simulink model "Auto_mode"  (R2016a)
settings: Solver=VariableStepAuto  StartTime=0.0  StopTime=50  FixedStep=Ts  RelTol=1e-3
model workspace (MAT data in the model file):
  AC_ATTITUDE_ACCEL_Y_CONTROLLER_MAX_RADSS = Simulink.Signal
  AC_ATTITUDE_ACCEL_Y_CONTROLLER_MAX_RADSS.DataType = 'double'
  AC_ATTITUDE_ACCEL_Y_CONTROLLER_MAX_RADSS.Dimensions = 1
  AC_ATTITUDE_ACCEL_Y_CONTROLLER_MAX_RADSS.DimensionsMode = 'auto'
  AC_ATTITUDE_ACCEL_Y_CONTROLLER_MAX_RADSS.Complexity = 'real'
  AC_ATTITUDE_ACCEL_Y_CONTROLLER_MAX_RADSS.SampleTime = -1
  AC_ATTITUDE_ACCEL_Y_CONTROLLER_MAX_RADSS.SamplingMode = 'Sample based'
  AC_ATTITUDE_ACCEL_Y_CONTROLLER_MAX_RADSS.InitialValue = '0.5'
  AC_ATTITUDE_CONTROL_MAX = Simulink.Signal
  AC_ATTITUDE_CONTROL_MAX.DataType = 'double'
  AC_ATTITUDE_CONTROL_MAX.Dimensions = 1
  AC_ATTITUDE_CONTROL_MAX.DimensionsMode = 'auto'
  AC_ATTITUDE_CONTROL_MAX.Complexity = 'real'
  AC_ATTITUDE_CONTROL_MAX.SampleTime = -1
  AC_ATTITUDE_CONTROL_MAX.SamplingMode = 'Sample based'
  AC_ATTITUDE_CONTROL_MAX.InitialValue = '0.5'
  AC_ATTITUDE_THRUST_ERROR_ANGLE = Simulink.Signal
  AC_ATTITUDE_THRUST_ERROR_ANGLE.DataType = 'double'
  AC_ATTITUDE_THRUST_ERROR_ANGLE.Dimensions = 1
  AC_ATTITUDE_THRUST_ERROR_ANGLE.DimensionsMode = 'auto'
  AC_ATTITUDE_THRUST_ERROR_ANGLE.Complexity = 'real'
  AC_ATTITUDE_THRUST_ERROR_ANGLE.SampleTime = -1
  AC_ATTITUDE_THRUST_ERROR_ANGLE.SamplingMode = 'Sample based'
  AC_ATTITUDE_THRUST_ERROR_ANGLE.InitialValue = '1000'
  ROLL_PITCH_INPUT_MAX = Simulink.Signal
  ROLL_PITCH_INPUT_MAX.DataType = 'double'
  ROLL_PITCH_INPUT_MAX.Dimensions = 1
  ROLL_PITCH_INPUT_MAX.DimensionsMode = 'auto'
  ROLL_PITCH_INPUT_MAX.Complexity = 'real'
  ROLL_PITCH_INPUT_MAX.SampleTime = -1
  ROLL_PITCH_INPUT_MAX.SamplingMode = 'Sample based'
  ROLL_PITCH_INPUT_MAX.InitialValue = '3000'
  Sig = Simulink.Signal
  Sig.DataType = 'auto'
  Sig.Dimensions = -1
  Sig.DimensionsMode = 'auto'
  Sig.Complexity = 'auto'
  Sig.SampleTime = -1
  Sig.SamplingMode = 'auto'
  Sig1 = Simulink.Signal
  Sig1.DataType = 'auto'
  Sig1.Dimensions = -1
  Sig1.DimensionsMode = 'auto'
  Sig1.Complexity = 'auto'
  Sig1.SampleTime = -1
  Sig1.SamplingMode = 'auto'
  acro_yaw_p = Simulink.Signal
  acro_yaw_p.DataType = 'double'
  acro_yaw_p.Dimensions = 1
  acro_yaw_p.DimensionsMode = 'auto'
  acro_yaw_p.Complexity = 'real'
  acro_yaw_p.SampleTime = -1
  acro_yaw_p.SamplingMode = 'Sample based'
  acro_yaw_p.InitialValue = '45'
  angle_max = Simulink.Signal
  angle_max.DataType = 'double'
  angle_max.Dimensions = 1
  angle_max.DimensionsMode = 'auto'
  angle_max.Complexity = 'real'
  angle_max.SampleTime = -1
  angle_max.SamplingMode = 'Sample based'
  angle_max.InitialValue = '3000'
  attitude_target_ang_vel = Simulink.Signal
  attitude_target_ang_vel.DataType = 'double'
  attitude_target_ang_vel.Dimensions = 3
  attitude_target_ang_vel.DimensionsMode = 'auto'
  attitude_target_ang_vel.Complexity = 'real'
  attitude_target_ang_vel.SampleTime = -1
  attitude_target_ang_vel.SamplingMode = 'Sample based'
  attitude_target_ang_vel.InitialValue = '[0 0 0]'
  attitude_target_euler_angle_x = Simulink.Signal
  attitude_target_euler_angle_x.DataType = 'double'
  attitude_target_euler_angle_x.Dimensions = 1
  attitude_target_euler_angle_x.DimensionsMode = 'auto'
  attitude_target_euler_angle_x.Complexity = 'real'
  attitude_target_euler_angle_x.SampleTime = -1
  attitude_target_euler_angle_x.SamplingMode = 'Sample based'
  attitude_target_euler_angle_x.InitialValue = '0'
  attitude_target_euler_angle_y = Simulink.Signal
  attitude_target_euler_angle_y.DataType = 'double'
  attitude_target_euler_angle_y.Dimensions = 1
  attitude_target_euler_angle_y.DimensionsMode = 'auto'
  attitude_target_euler_angle_y.Complexity = 'real'
  attitude_target_euler_angle_y.SampleTime = -1
  attitude_target_euler_angle_y.SamplingMode = 'Sample based'
  attitude_target_euler_angle_y.InitialValue = '0'
  attitude_target_euler_angle_z = Simulink.Signal
  attitude_target_euler_angle_z.DataType = 'double'
  attitude_target_euler_angle_z.Dimensions = 1
  attitude_target_euler_angle_z.DimensionsMode = 'auto'
  attitude_target_euler_angle_z.Complexity = 'real'
  attitude_target_euler_angle_z.SampleTime = -1
  attitude_target_euler_angle_z.SamplingMode = 'Sample based'
  attitude_target_euler_angle_z.InitialValue = '0'
  attitude_target_euler_rate = Simulink.Signal
  attitude_target_euler_rate.DataType = 'double'
  attitude_target_euler_rate.Dimensions = 3
  attitude_target_euler_rate.DimensionsMode = 'auto'
  attitude_target_euler_rate.Complexity = 'real'
  attitude_target_euler_rate.SampleTime = -1
  attitude_target_euler_rate.SamplingMode = 'Sample based'
  attitude_target_euler_rate.InitialValue = '[0 0 0]'
  attitude_target_quat = Simulink.Signal
  attitude_target_quat.DataType = 'double'
  attitude_target_quat.Dimensions = 4
  attitude_target_quat.DimensionsMode = 'auto'
  attitude_target_quat.Complexity = 'real'
  attitude_target_quat.SampleTime = -1
  attitude_target_quat.SamplingMode = 'Sample based'
  attitude_target_quat.InitialValue = '[1 0 0 0]'
  attitude_vehicle_quat = Simulink.Signal
  attitude_vehicle_quat.DataType = 'double'
  attitude_vehicle_quat.Dimensions = 4
  attitude_vehicle_quat.DimensionsMode = 'auto'
  attitude_vehicle_quat.Complexity = 'real'
  attitude_vehicle_quat.SampleTime = -1
  attitude_vehicle_quat.SamplingMode = 'Sample based'
  attitude_vehicle_quat.InitialValue = '[1 0 0 0]'
  dt = Simulink.Signal
  dt.DataType = 'double'
  dt.Dimensions = 1
  dt.DimensionsMode = 'auto'
  dt.Complexity = 'real'
  dt.SampleTime = -1
  dt.SamplingMode = 'Sample based'
  dt.InitialValue = '0.01'
  false = 0
  limit_roll_pitch = Simulink.Signal
  limit_roll_pitch.DataType = 'double'
  limit_roll_pitch.Dimensions = 1
  limit_roll_pitch.DimensionsMode = 'auto'
  limit_roll_pitch.Complexity = 'real'
  limit_roll_pitch.SampleTime = -1
  limit_roll_pitch.SamplingMode = 'Sample based'
  limit_roll_pitch.InitialValue = '0.0'
  limit_throttle_upper = Simulink.Signal
  limit_throttle_upper.DataType = 'logical'
  limit_throttle_upper.Dimensions = 1
  limit_throttle_upper.DimensionsMode = 'auto'
  limit_throttle_upper.Complexity = 'real'
  limit_throttle_upper.SampleTime = -1
  limit_throttle_upper.SamplingMode = 'Sample based'
  limit_throttle_upper.InitialValue = '0'
  limit_yaw = Simulink.Signal
  limit_yaw.DataType = 'double'
  limit_yaw.Dimensions = 1
  limit_yaw.DimensionsMode = 'auto'
  limit_yaw.Complexity = 'real'
  limit_yaw.SampleTime = -1
  limit_yaw.SamplingMode = 'Sample based'
  limit_yaw.InitialValue = '0'
  loop_rate = Simulink.Signal
  loop_rate.DataType = 'double'
  loop_rate.Dimensions = 1
  loop_rate.DimensionsMode = 'auto'
  loop_rate.Complexity = 'real'
  loop_rate.SampleTime = -1
  loop_rate.SamplingMode = 'Sample based'
  loop_rate.InitialValue = '100'
  pitch_attitude_kP = Simulink.Signal
  pitch_attitude_kP.DataType = 'double'
  pitch_attitude_kP.Dimensions = 1
  pitch_attitude_kP.DimensionsMode = 'auto'
  pitch_attitude_kP.Complexity = 'real'
  pitch_attitude_kP.SampleTime = -1
  pitch_attitude_kP.SamplingMode = 'Sample based'
  pitch_attitude_kP.InitialValue = '20'
  pitch_factor = Simulink.Signal
  pitch_factor.DataType = 'double'
  pitch_factor.Dimensions = 4
  pitch_factor.DimensionsMode = 'auto'
  pitch_factor.Complexity = 'real'
  pitch_factor.SampleTime = -1
  pitch_factor.SamplingMode = 'Sample based'
  pitch_factor.InitialValue = '[cos(deg2rad(15)) -cos(deg2rad(15)) cos(deg2rad(15)) -cos(deg2rad(15))]'
  pitch_rate_derivative = Simulink.Signal
  pitch_rate_derivative.DataType = 'double'
  pitch_rate_derivative.Dimensions = 1
  pitch_rate_derivative.DimensionsMode = 'auto'
  pitch_rate_derivative.Complexity = 'real'
  pitch_rate_derivative.SampleTime = -1
  pitch_rate_derivative.SamplingMode = 'Sample based'
  pitch_rate_derivative.InitialValue = '0'
  pitch_rate_error_rads = Simulink.Signal
  pitch_rate_error_rads.DataType = 'double'
  pitch_rate_error_rads.Dimensions = 1
  pitch_rate_error_rads.DimensionsMode = 'auto'
  pitch_rate_error_rads.Complexity = 'real'
  pitch_rate_error_rads.SampleTime = -1
  pitch_rate_error_rads.SamplingMode = 'Sample based'
  pitch_rate_error_rads.InitialValue = '0'
  pitch_rate_filt_hz = Simulink.Signal
  pitch_rate_filt_hz.DataType = 'double'
  pitch_rate_filt_hz.Dimensions = 1
  pitch_rate_filt_hz.DimensionsMode = 'auto'
  pitch_rate_filt_hz.Complexity = 'real'
  pitch_rate_filt_hz.SampleTime = -1
  pitch_rate_filt_hz.SamplingMode = 'Sample based'
  pitch_rate_filt_hz.InitialValue = '1/(2*pi)'
  pitch_rate_imax = Simulink.Signal
  pitch_rate_imax.DataType = 'double'
  pitch_rate_imax.Dimensions = 1
  pitch_rate_imax.DimensionsMode = 'auto'
  pitch_rate_imax.Complexity = 'real'
  pitch_rate_imax.SampleTime = -1
  pitch_rate_imax.SamplingMode = 'Sample based'
  pitch_rate_imax.InitialValue = '200'
  pitch_rate_integrator = Simulink.Signal
  pitch_rate_integrator.DataType = 'double'
  pitch_rate_integrator.Dimensions = 1
  pitch_rate_integrator.DimensionsMode = 'auto'
  pitch_rate_integrator.Complexity = 'real'
  pitch_rate_integrator.SampleTime = -1
  pitch_rate_integrator.SamplingMode = 'Sample based'
  pitch_rate_integrator.InitialValue = '0'
  pitch_rate_kD = Simulink.Signal
  pitch_rate_kD.DataType = 'double'
  pitch_rate_kD.Dimensions = 1
  pitch_rate_kD.DimensionsMode = 'auto'
  pitch_rate_kD.Complexity = 'real'
  pitch_rate_kD.SampleTime = -1
  pitch_rate_kD.SamplingMode = 'Sample based'
  pitch_rate_kD.InitialValue = '0.004'
  pitch_rate_kI = Simulink.Signal
  pitch_rate_kI.DataType = 'double'
  pitch_rate_kI.Dimensions = 1
  pitch_rate_kI.DimensionsMode = 'auto'
  pitch_rate_kI.Complexity = 'real'
  pitch_rate_kI.SampleTime = -1
  pitch_rate_kI.SamplingMode = 'Sample based'
  pitch_rate_kI.InitialValue = '0.1'
  pitch_rate_kP = Simulink.Signal
  pitch_rate_kP.DataType = 'double'
  pitch_rate_kP.Dimensions = 1
  pitch_rate_kP.DimensionsMode = 'auto'
  pitch_rate_kP.Complexity = 'real'
  pitch_rate_kP.SampleTime = -1
  pitch_rate_kP.SamplingMode = 'Sample based'
  pitch_rate_kP.InitialValue = '0.5'
  pitch_rate_last_input = Simulink.Signal
  pitch_rate_last_input.DataType = 'double'
  pitch_rate_last_input.Dimensions = 1
  pitch_rate_last_input.DimensionsMode = 'auto'
  pitch_rate_last_input.Complexity = 'real'
  pitch_rate_last_input.SampleTime = -1
  pitch_rate_last_input.SamplingMode = 'Sample based'
  pitch_rate_last_input.InitialValue = '0'
  pitch_rate_proportional = Simulink.Signal
  pitch_rate_proportional.DataType = 'double'
  pitch_rate_proportional.Dimensions = 1
  pitch_rate_proportional.DimensionsMode = 'auto'
  pitch_rate_proportional.Complexity = 'real'
  pitch_rate_proportional.SampleTime = -1
  pitch_rate_proportional.SamplingMode = 'Sample based'
  pitch_rate_proportional.InitialValue = '0'
  pwm_max = Simulink.Signal
  pwm_max.DataType = 'double'
  pwm_max.Dimensions = 1
  pwm_max.DimensionsMode = 'auto'
  pwm_max.Complexity = 'real'
  pwm_max.SampleTime = -1
  pwm_max.SamplingMode = 'Sample based'
  pwm_max.InitialValue = '2000'
  pwm_min = Simulink.Signal
  pwm_min.DataType = 'double'
  pwm_min.Dimensions = 1
  pwm_min.DimensionsMode = 'auto'
  pwm_min.Complexity = 'real'
  pwm_min.SampleTime = -1
  pwm_min.SamplingMode = 'Sample based'
  pwm_min.InitialValue = '1039'
  rate_bf_ff_enabled = Simulink.Signal
  rate_bf_ff_enabled.DataType = 'double'
  rate_bf_ff_enabled.Dimensions = 1
  rate_bf_ff_enabled.DimensionsMode = 'auto'
  rate_bf_ff_enabled.Complexity = 'real'
  rate_bf_ff_enabled.SampleTime = -1
  rate_bf_ff_enabled.SamplingMode = 'Sample based'
  rate_bf_ff_enabled.InitialValue = '0'
  rate_target_ang_vel = Simulink.Signal
  rate_target_ang_vel.DataType = 'double'
  rate_target_ang_vel.Dimensions = 3
  rate_target_ang_vel.DimensionsMode = 'auto'
  rate_target_ang_vel.Complexity = 'real'
  rate_target_ang_vel.SampleTime = -1
  rate_target_ang_vel.SamplingMode = 'Sample based'
  rate_target_ang_vel.InitialValue = '[0 0 0]'
  roll_attitude_kP = Simulink.Signal
  roll_attitude_kP.DataType = 'double'
  roll_attitude_kP.Dimensions = 1
  roll_attitude_kP.DimensionsMode = 'auto'
  roll_attitude_kP.Complexity = 'real'
  roll_attitude_kP.SampleTime = -1
  roll_attitude_kP.SamplingMode = 'Sample based'
  roll_attitude_kP.InitialValue = '20'
  roll_factor = Simulink.Signal
  roll_factor.DataType = 'double'
  roll_factor.Dimensions = 4
  roll_factor.DimensionsMode = 'auto'
  roll_factor.Complexity = 'real'
  roll_factor.SampleTime = -1
  roll_factor.SamplingMode = 'Sample based'
  roll_factor.InitialValue = '[-sin(deg2rad(15)) sin(deg2rad(15)) sin(deg2rad(15)) -sin(deg2rad(15))]'
  roll_rate_derivative = Simulink.Signal
  roll_rate_derivative.DataType = 'double'
  roll_rate_derivative.Dimensions = 1
  roll_rate_derivative.DimensionsMode = 'auto'
  roll_rate_derivative.Complexity = 'real'
  roll_rate_derivative.SampleTime = -1
  roll_rate_derivative.SamplingMode = 'Sample based'
  roll_rate_derivative.InitialValue = '0'
  roll_rate_error_rads = Simulink.Signal
  roll_rate_error_rads.DataType = 'double'
  roll_rate_error_rads.Dimensions = 1
  roll_rate_error_rads.DimensionsMode = 'auto'
  roll_rate_error_rads.Complexity = 'real'
  roll_rate_error_rads.SampleTime = -1
  roll_rate_error_rads.SamplingMode = 'Sample based'
  roll_rate_error_rads.InitialValue = '0'
  roll_rate_filt_hz = Simulink.Signal
  roll_rate_filt_hz.DataType = 'double'
  roll_rate_filt_hz.Dimensions = 1
  roll_rate_filt_hz.DimensionsMode = 'auto'
  roll_rate_filt_hz.Complexity = 'real'
  roll_rate_filt_hz.SampleTime = -1
  roll_rate_filt_hz.SamplingMode = 'Sample based'
  roll_rate_filt_hz.InitialValue = '1/(2*pi)'
  roll_rate_imax = Simulink.Signal
  roll_rate_imax.DataType = 'double'
  roll_rate_imax.Dimensions = 1
  roll_rate_imax.DimensionsMode = 'auto'
  roll_rate_imax.Complexity = 'real'
  roll_rate_imax.SampleTime = -1
  roll_rate_imax.SamplingMode = 'Sample based'
  roll_rate_imax.InitialValue = '200'
  roll_rate_integrator = Simulink.Signal
  roll_rate_integrator.DataType = 'double'
  roll_rate_integrator.Dimensions = 1
  roll_rate_integrator.DimensionsMode = 'auto'
  roll_rate_integrator.Complexity = 'real'
  roll_rate_integrator.SampleTime = -1
  roll_rate_integrator.SamplingMode = 'Sample based'
  roll_rate_integrator.InitialValue = '0'
  roll_rate_kD = Simulink.Signal
  roll_rate_kD.DataType = 'double'
  roll_rate_kD.Dimensions = 1
  roll_rate_kD.DimensionsMode = 'auto'
  roll_rate_kD.Complexity = 'real'
  roll_rate_kD.SampleTime = -1
  roll_rate_kD.SamplingMode = 'Sample based'
  roll_rate_kD.InitialValue = '0.004'
  roll_rate_kI = Simulink.Signal
  roll_rate_kI.DataType = 'double'
  roll_rate_kI.Dimensions = 1
  roll_rate_kI.DimensionsMode = 'auto'
  roll_rate_kI.Complexity = 'real'
  roll_rate_kI.SampleTime = -1
  roll_rate_kI.SamplingMode = 'Sample based'
  roll_rate_kI.InitialValue = '0.1'
  roll_rate_kP = Simulink.Signal
  roll_rate_kP.DataType = 'double'
  roll_rate_kP.Dimensions = 1
  roll_rate_kP.DimensionsMode = 'auto'
  roll_rate_kP.Complexity = 'real'
  roll_rate_kP.SampleTime = -1
  roll_rate_kP.SamplingMode = 'Sample based'
  roll_rate_kP.InitialValue = '1'
  roll_rate_last_input = Simulink.Signal
  roll_rate_last_input.DataType = 'double'
  roll_rate_last_input.Dimensions = 1
  roll_rate_last_input.DimensionsMode = 'auto'
  roll_rate_last_input.Complexity = 'real'
  roll_rate_last_input.SampleTime = -1
  roll_rate_last_input.SamplingMode = 'Sample based'
  roll_rate_last_input.InitialValue = '0'
  roll_rate_proportional = Simulink.Signal
  roll_rate_proportional.DataType = 'double'
  roll_rate_proportional.Dimensions = 1
  roll_rate_proportional.DimensionsMode = 'auto'
  roll_rate_proportional.Complexity = 'real'
  roll_rate_proportional.SampleTime = -1
  roll_rate_proportional.SamplingMode = 'Sample based'
  roll_rate_proportional.InitialValue = '0'
  spin_max = Simulink.Signal
  spin_max.DataType = 'double'
  spin_max.Dimensions = 1
  spin_max.DimensionsMode = 'auto'
  spin_max.Complexity = 'real'
  spin_max.SampleTime = -1
  spin_max.SamplingMode = 'Sample based'
  spin_max.InitialValue = '0.95'
  spin_min = Simulink.Signal
  spin_min.DataType = 'double'
  spin_min.Dimensions = 1
  spin_min.DimensionsMode = 'auto'
  spin_min.Complexity = 'real'
  spin_min.SampleTime = -1
  spin_min.SamplingMode = 'Sample based'
  spin_min.InitialValue = '0.15'
  throttle_avg_max = Simulink.Signal
  throttle_avg_max.DataType = 'double'
  throttle_avg_max.Dimensions = 1
  throttle_avg_max.DimensionsMode = 'auto'
  throttle_avg_max.Complexity = 'real'
  throttle_avg_max.SampleTime = -1
  throttle_avg_max.SamplingMode = 'Sample based'
  throttle_avg_max.InitialValue = '0'
  throttle_filter_cutoff_freq = Simulink.Signal
  throttle_filter_cutoff_freq.DataType = 'double'
  throttle_filter_cutoff_freq.Dimensions = 1
  throttle_filter_cutoff_freq.DimensionsMode = 'auto'
  throttle_filter_cutoff_freq.Complexity = 'real'
  throttle_filter_cutoff_freq.SampleTime = -1
  throttle_filter_cutoff_freq.SamplingMode = 'Sample based'
  throttle_filter_cutoff_freq.InitialValue = '0.5'
  throttle_filter_output = Simulink.Signal
  throttle_filter_output.DataType = 'double'
  throttle_filter_output.Dimensions = 1
  throttle_filter_output.DimensionsMode = 'auto'
  throttle_filter_output.Complexity = 'real'
  throttle_filter_output.SampleTime = -1
  throttle_filter_output.SamplingMode = 'Sample based'
  throttle_filter_output.InitialValue = '0'
  throttle_in = Simulink.Signal
  throttle_in.DataType = 'double'
  throttle_in.Dimensions = 1
  throttle_in.DimensionsMode = 'auto'
  throttle_in.Complexity = 'real'
  throttle_in.SampleTime = -1
  throttle_in.SamplingMode = 'Sample based'
  throttle_in.InitialValue = '0'
  throttle_rpy_mix = Simulink.Signal
  throttle_rpy_mix.DataType = 'double'
  throttle_rpy_mix.Dimensions = 1
  throttle_rpy_mix.DimensionsMode = 'auto'
  throttle_rpy_mix.Complexity = 'real'
  throttle_rpy_mix.SampleTime = -1
  throttle_rpy_mix.SamplingMode = 'Sample based'
  throttle_rpy_mix.InitialValue = '0'
  throttle_rpy_mix_desired = Simulink.Signal
  throttle_rpy_mix_desired.DataType = 'double'
  throttle_rpy_mix_desired.Dimensions = 1
  throttle_rpy_mix_desired.DimensionsMode = 'auto'
  throttle_rpy_mix_desired.Complexity = 'real'
  throttle_rpy_mix_desired.SampleTime = -1
  throttle_rpy_mix_desired.SamplingMode = 'Sample based'
  throttle_rpy_mix_desired.InitialValue = '0'
  throttle_thrust = Simulink.Signal
  throttle_thrust.DataType = 'double'
  throttle_thrust.Dimensions = 1
  throttle_thrust.DimensionsMode = 'auto'
  throttle_thrust.Complexity = 'real'
  throttle_thrust.SampleTime = -1
  throttle_thrust.SamplingMode = 'Sample based'
  throttle_thrust.InitialValue = '0'
  throttle_thrust_best_rpy = Simulink.Signal
  throttle_thrust_best_rpy.DataType = 'double'
  throttle_thrust_best_rpy.Dimensions = 1
  throttle_thrust_best_rpy.DimensionsMode = 'auto'
  throttle_thrust_best_rpy.Complexity = 'real'
  throttle_thrust_best_rpy.SampleTime = -1
  throttle_thrust_best_rpy.SamplingMode = 'Sample based'
  throttle_thrust_best_rpy.InitialValue = '0'
  throttle_thrust_max = Simulink.Signal
  throttle_thrust_max.DataType = 'double'
  throttle_thrust_max.Dimensions = 1
  throttle_thrust_max.DimensionsMode = 'auto'
  throttle_thrust_max.Complexity = 'real'
  throttle_thrust_max.SampleTime = -1
  throttle_thrust_max.SamplingMode = 'Sample based'
  throttle_thrust_max.InitialValue = '1'
  thrust_error_angle = Simulink.Signal
  thrust_error_angle.DataType = 'double'
  thrust_error_angle.Dimensions = 1
  thrust_error_angle.DimensionsMode = 'auto'
  thrust_error_angle.Complexity = 'real'
  thrust_error_angle.SampleTime = -1
  thrust_error_angle.SamplingMode = 'Sample based'
  thrust_error_angle.InitialValue = '0'
  thrust_rpyt_out = Simulink.Signal
  thrust_rpyt_out.DataType = 'double'
  thrust_rpyt_out.Dimensions = 4
  thrust_rpyt_out.DimensionsMode = 'auto'
  thrust_rpyt_out.Complexity = 'real'
  thrust_rpyt_out.SampleTime = -1
  thrust_rpyt_out.SamplingMode = 'Sample based'
  thrust_rpyt_out.InitialValue = '[0 0 0 0]'
  true = 1
  use_ff_and_input_shaping = Simulink.Signal
  use_ff_and_input_shaping.DataType = 'double'
  use_ff_and_input_shaping.Dimensions = 1
  use_ff_and_input_shaping.DimensionsMode = 'auto'
  use_ff_and_input_shaping.Complexity = 'real'
  use_ff_and_input_shaping.SampleTime = -1
  use_ff_and_input_shaping.SamplingMode = 'Sample based'
  use_ff_and_input_shaping.InitialValue = '0'
  variableType = 'S'
  yaw_allowed = Simulink.Signal
  yaw_allowed.DataType = 'double'
  yaw_allowed.Dimensions = 1
  yaw_allowed.DimensionsMode = 'auto'
  yaw_allowed.Complexity = 'real'
  yaw_allowed.SampleTime = -1
  yaw_allowed.SamplingMode = 'Sample based'
  yaw_allowed.InitialValue = '1'
  yaw_attitude_kP = Simulink.Signal
  yaw_attitude_kP.DataType = 'double'
  yaw_attitude_kP.Dimensions = 1
  yaw_attitude_kP.DimensionsMode = 'auto'
  yaw_attitude_kP.Complexity = 'real'
  yaw_attitude_kP.SampleTime = -1
  yaw_attitude_kP.SamplingMode = 'Sample based'
  yaw_attitude_kP.InitialValue = '4.5'
  yaw_factor = Simulink.Signal
  yaw_factor.DataType = 'double'
  yaw_factor.Dimensions = 4
  yaw_factor.DimensionsMode = 'auto'
  yaw_factor.Complexity = 'real'
  yaw_factor.SampleTime = -1
  yaw_factor.SamplingMode = 'Sample based'
  yaw_factor.InitialValue = '[0.1 0.1 -0.1 -0.1]'
  yaw_headroom = Simulink.Signal
  yaw_headroom.DataType = 'double'
  yaw_headroom.Dimensions = 1
  yaw_headroom.DimensionsMode = 'auto'
  yaw_headroom.Complexity = 'real'
  yaw_headroom.SampleTime = -1
  yaw_headroom.SamplingMode = 'Sample based'
  yaw_headroom.InitialValue = '200'
  yaw_rate_derivative = Simulink.Signal
  yaw_rate_derivative.DataType = 'double'
  yaw_rate_derivative.Dimensions = 1
  yaw_rate_derivative.DimensionsMode = 'auto'
  yaw_rate_derivative.Complexity = 'real'
  yaw_rate_derivative.SampleTime = -1
  yaw_rate_derivative.SamplingMode = 'Sample based'
  yaw_rate_derivative.InitialValue = '0'
  yaw_rate_error_rads = Simulink.Signal
  yaw_rate_error_rads.DataType = 'double'
  yaw_rate_error_rads.Dimensions = 1
  yaw_rate_error_rads.DimensionsMode = 'auto'
  yaw_rate_error_rads.Complexity = 'real'
  yaw_rate_error_rads.SampleTime = -1
  yaw_rate_error_rads.SamplingMode = 'Sample based'
  yaw_rate_error_rads.InitialValue = '0'
  yaw_rate_filt_hz = Simulink.Signal
  yaw_rate_filt_hz.DataType = 'double'
  yaw_rate_filt_hz.Dimensions = 1
  yaw_rate_filt_hz.DimensionsMode = 'auto'
  yaw_rate_filt_hz.Complexity = 'real'
  yaw_rate_filt_hz.SampleTime = -1
  yaw_rate_filt_hz.SamplingMode = 'Sample based'
  yaw_rate_filt_hz.InitialValue = '1/(2*pi)'
  yaw_rate_imax = Simulink.Signal
  yaw_rate_imax.DataType = 'double'
  yaw_rate_imax.Dimensions = 1
  yaw_rate_imax.DimensionsMode = 'auto'
  yaw_rate_imax.Complexity = 'real'
  yaw_rate_imax.SampleTime = -1
  yaw_rate_imax.SamplingMode = 'Sample based'
  yaw_rate_imax.InitialValue = '200'
  yaw_rate_integrator = Simulink.Signal
  yaw_rate_integrator.DataType = 'double'
  yaw_rate_integrator.Dimensions = 1
  yaw_rate_integrator.DimensionsMode = 'auto'
  yaw_rate_integrator.Complexity = 'real'
  yaw_rate_integrator.SampleTime = -1
  yaw_rate_integrator.SamplingMode = 'Sample based'
  yaw_rate_integrator.InitialValue = '0'
  yaw_rate_kD = Simulink.Signal
  yaw_rate_kD.DataType = 'double'
  yaw_rate_kD.Dimensions = 1
  yaw_rate_kD.DimensionsMode = 'auto'
  yaw_rate_kD.Complexity = 'real'
  yaw_rate_kD.SampleTime = -1
  yaw_rate_kD.SamplingMode = 'Sample based'
  yaw_rate_kD.InitialValue = '5'
  yaw_rate_kI = Simulink.Signal
  yaw_rate_kI.DataType = 'double'
  yaw_rate_kI.Dimensions = 1
  yaw_rate_kI.DimensionsMode = 'auto'
  yaw_rate_kI.Complexity = 'real'
  yaw_rate_kI.SampleTime = -1
  yaw_rate_kI.SamplingMode = 'Sample based'
  yaw_rate_kI.InitialValue = '0.1'
  yaw_rate_kP = Simulink.Signal
  yaw_rate_kP.DataType = 'double'
  yaw_rate_kP.Dimensions = 1
  yaw_rate_kP.DimensionsMode = 'auto'
  yaw_rate_kP.Complexity = 'real'
  yaw_rate_kP.SampleTime = -1
  yaw_rate_kP.SamplingMode = 'Sample based'
  yaw_rate_kP.InitialValue = '0.2'
  yaw_rate_last_input = Simulink.Signal
  yaw_rate_last_input.DataType = 'double'
  yaw_rate_last_input.Dimensions = 1
  yaw_rate_last_input.DimensionsMode = 'auto'
  yaw_rate_last_input.Complexity = 'real'
  yaw_rate_last_input.SampleTime = -1
  yaw_rate_last_input.SamplingMode = 'Sample based'
  yaw_rate_last_input.InitialValue = '0'
  yaw_rate_proportional = Simulink.Signal
  yaw_rate_proportional.DataType = 'double'
  yaw_rate_proportional.Dimensions = 1
  yaw_rate_proportional.DimensionsMode = 'auto'
  yaw_rate_proportional.Complexity = 'real'
  yaw_rate_proportional.SampleTime = -1
  yaw_rate_proportional.SamplingMode = 'Sample based'
  yaw_rate_proportional.InitialValue = '0'
undefined symbols (not defined in the file): Ts
libraries: aerolibactuator x2, vrlib x2, aerolib6dof2 x1, aerolibutil x1, aerolibconvert2 x1
settings Model: Creator=s121814  LastModifiedBy=GusBus
settings SolverCC: ZeroCrossControl=DisableAll
settings DataIOCC: SaveFormat=Array  SaveState=on

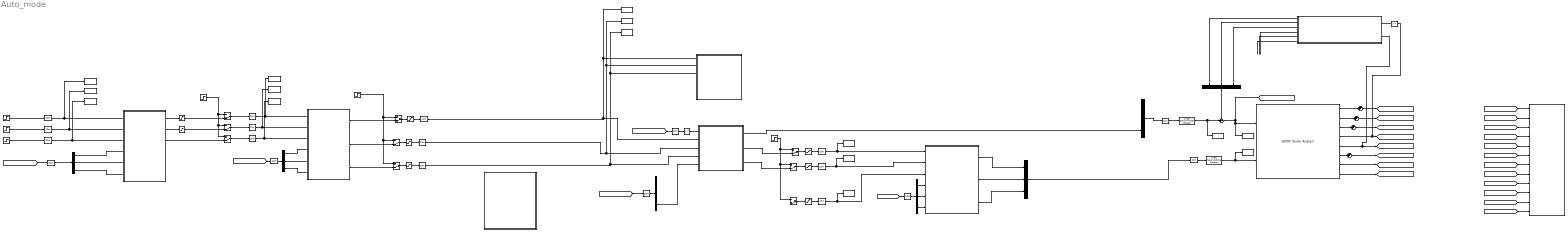
== system Auto_mode ==
  note: Step Response and Switches used for tuning
  Demux{,1..3} (4 alike) : Demux  Outputs=3
  Flight Kinematics : aerolib6dof2/6DOF (Euler Angles)  units=Metric (MKS)  mtype=Fixed  rep=Euler Angles  xme_0=[0 0 0]  Vm_0=[0 0 0]  eul_0=[0 0 0]  pm_0=[0 0 0]  mass_0=3.352  mass_e=0.5  mass_f=2.0  inertia=[0.025028 0 0; 0 0.16926 0; 0 0 0.170197]  inertia_e=eye(3)  inertia_f=2*eye(3)  k_quat=1.0  vre_flag=on
  Gravity and Drag Distrubance Calculation : MATLAB Function  TreatAsAtomicUnit=on
  Linear Second-Order Actuator1 : aerolibactuator/Linear Second-Order Actuator  wn_fin=100  z_fin=1  fin_act_0=0  fin_act_vel=0
  Linear Second-Order Actuator2 : aerolibactuator/Linear Second-Order Actuator  wn_fin=100  z_fin=1  fin_act_0=0  fin_act_vel=0
  Linear Velocity Controller : Subsystem
  Manual Switch{,1..5,9..11} (9 alike) : ManualSwitch  CurrentSetting=0
  Math Function : Math  Operator=transpose  SaturateOnIntegerOverflow=on
  Math Function1 : Math  Operator=transpose  SaturateOnIntegerOverflow=on
  Position Controller : Subsystem
  Rate Controller : Subsystem
  Saturation : Saturate  UpperLimit=deg2rad(15)  LowerLimit=-deg2rad(15)
  Saturation1 : Saturate  UpperLimit=deg2rad(15)  LowerLimit=-deg2rad(15)
  Saturation2 : Saturate  UpperLimit=15  LowerLimit=-15
  Saturation3 : Saturate  UpperLimit=15  LowerLimit=-15
  Saturation4 : Saturate  UpperLimit=100  LowerLimit=-100
  Saturation5 : Saturate  UpperLimit=15  LowerLimit=-15
  Saturation6 : Saturate  UpperLimit=1  LowerLimit=-1
  Saturation7 : Saturate  UpperLimit=1  LowerLimit=-1
  Step : Step  Time=0  After=0  SampleTime=0
  Step1 : Step  Time=0  After=0  SampleTime=0
  Step2 : Step  After=0  SampleTime=0
  Step3 : Step  SampleTime=0
  Step5 : Step  After=0.18  SampleTime=0
  Step6 : Step  After=5  SampleTime=0
  Sum1 : Sum  Inputs=-+|
  Sum{5,7,9..10} (4 alike) : Sum  Inputs=++|
  Thrust Controller : Subsystem
  Tilt Angle Controller : Subsystem
  To Workspace and Graphics : Subsystem
  To Workspace1 : ToWorkspace  VariableName=refrollrate  SampleTime=-1
  To Workspace10 : ToWorkspace  VariableName=forces  SampleTime=-1
  To Workspace11 : ToWorkspace  VariableName=moments  SampleTime=-1
  To Workspace12 : ToWorkspace  VariableName=refxvel_e  SampleTime=-1
  To Workspace13 : ToWorkspace  VariableName=refyvel_e  SampleTime=-1
  To Workspace14 : ToWorkspace  VariableName=refzvel_e  SampleTime=-1
  To Workspace15 : ToWorkspace  VariableName=forces1  SampleTime=-1
  To Workspace2 : ToWorkspace  VariableName=refpitchrate  SampleTime=-1
  To Workspace3 : ToWorkspace  VariableName=refxaccel  SampleTime=-1
  To Workspace4 : ToWorkspace  VariableName=refyaccel  SampleTime=-1
  To Workspace5 : ToWorkspace  VariableName=refzaccel  SampleTime=-1
  To Workspace6 : ToWorkspace  VariableName=refyawrate  SampleTime=-1
  To Workspace7 : ToWorkspace  VariableName=refxpos  SampleTime=-1
  To Workspace8 : ToWorkspace  VariableName=refypos  SampleTime=-1
  To Workspace9 : ToWorkspace  VariableName=refzpos  SampleTime=-1
  Vector Concatenate1 : Concatenate  NumInputs=3
  Vector Concatenate2 : Concatenate  NumInputs=3
  Vector Concatenate7 : Concatenate  NumInputs=3
  Vector Rotation : Subsystem
  Zero-Order Hold{1..19} (19 alike) : ZeroOrderHold  SampleTime=Ts
  tag scope: body_forces=global, body_linear_acceleration=global, body_linear_velocity=global, body_rotational_acceleration=global, body_rotational_velocity=global, dcm_body_earth=global, earth_linear_position=global, earth_linear_velocity=global, euler_angles_rad=global
  wires:
  [body_rotational_velocity] -> To Workspace and Graphics/6(body_rotational_velocity)
  [body_linear_acceleration] -> To Workspace and Graphics/8(body_linear_acceleration)
  [body_rotational_acceleration] -> To Workspace and Graphics/7(body_rotational_acceleration)
  [body_linear_velocity] -> To Workspace and Graphics/5(body_linear_velocity)
  [dcm_body_earth] -> To Workspace and Graphics/4(dcm_body_earth)
  [euler_angles_rad] -> To Workspace and Graphics/3(euler_angles_rad)
  [earth_linear_position] -> To Workspace and Graphics/2(earth_linear_position)
  [earth_linear_velocity] -> To Workspace and Graphics/1(earth_linear_velocity)
  Sum7/1 -> [earth_linear_velocity]  "earth_linear_velocity"
  Flight Kinematics/7 -> [body_rotational_acceleration]  "body_rotational_acceleration"
  Flight Kinematics/8 -> [body_linear_acceleration]  "body_linear_acceleration"
  Vector Concatenate7/1 -> Zero-Order Hold5/1
  Sum10/1 -> [euler_angles_rad]
  Flight Kinematics/3 -> Sum10/2  "euler_angles_rad"
  Sum9/1 -> [earth_linear_position]
  Flight Kinematics/2 -> Sum9/2
  Flight Kinematics/6 -> Sum5/2  "body_rotational_velocity"
  Sum5/1 -> [body_rotational_velocity]
  Flight Kinematics/1 -> Sum7/2
  [earth_linear_position_est] -> To Workspace and Graphics/12(earth_linear_position_est)
  [earth_linear_velocity_est] -> To Workspace and Graphics/11(earth_linear_velocity_est)
  [body_rotational_velocity_est] -> To Workspace and Graphics/10(body_rotational_velocity_est)
  [euler_angles_rad_est] -> To Workspace and Graphics/9(euler_angles_rad_est)
  Rate Controller/1(Torque Phi) -> Vector Concatenate7/1
  Rate Controller/2(Torque Theta) -> Vector Concatenate7/2
  Rate Controller/3(Torque Psi) -> Vector Concatenate7/3
  Demux/1 -> Rate Controller/4(roll_rate_current)
  Demux/2 -> Rate Controller/5(pitch_rate_current)
  Demux/3 -> Rate Controller/6(yaw_rate_current)
  [body_rotational_velocity] -> Zero-Order Hold1/1
  Zero-Order Hold1/1 -> Demux/1
  Zero-Order Hold5/1 -> Linear Second-Order Actuator1/1
  Vector Concatenate1/1 -> Zero-Order Hold6/1
  Zero-Order Hold6/1 -> Linear Second-Order Actuator2/1
  Linear Second-Order Actuator1/1 -> To Workspace11/1, Flight Kinematics/2  "moments"
  Sum1/1 -> [body_forces], To Workspace10/1, Flight Kinematics/1  "Forces"
  Step/1 -> Zero-Order Hold2/1  "x_pos_target"
  Step2/1 -> Zero-Order Hold4/1  "z_pos_target"
  Step1/1 -> Zero-Order Hold3/1  "y_pos_target"
  Zero-Order Hold2/1 -> To Workspace7/1, Position Controller/1(x_pos_target)
  Zero-Order Hold3/1 -> To Workspace8/1, Position Controller/2(y_pos_target)
  Zero-Order Hold4/1 -> To Workspace9/1, Position Controller/3(z_pos_target)
  [earth_linear_position] -> Zero-Order Hold14/1
  Demux2/2 -> Position Controller/5(y_pos_current)
  Demux2/1 -> Position Controller/4(x_pos_current)
  Demux2/3 -> Position Controller/6(z_pos_current)
  Saturation/1 -> Zero-Order Hold8/1
  Saturation1/1 -> Zero-Order Hold9/1
  Saturation2/1 -> Zero-Order Hold19/1
  Saturation3/1 -> Zero-Order Hold18/1
  Saturation4/1 -> Zero-Order Hold17/1
  [dcm_body_earth] -> Zero-Order Hold16/1
  Saturation5/1 -> Zero-Order Hold10/1
  Zero-Order Hold14/1 -> Demux2/1
  Zero-Order Hold16/1 -> Math Function/1
  Step3/1 -> Manual Switch2/1, Manual Switch/1, Manual Switch1/1
  Manual Switch/1 -> Saturation3/1
  Manual Switch1/1 -> Saturation2/1
  Manual Switch2/1 -> Saturation4/1
  Linear Velocity Controller/1(x_accel_desired_earth) -> Manual Switch1/2
  Linear Velocity Controller/2(y_accel_desired_earth) -> Manual Switch/2
  Linear Velocity Controller/3(z_accel_desired_earth) -> Manual Switch2/2
  Tilt Angle Controller/3(desired_pitch_rate_rad/s) -> Manual Switch3/2
  Math Function/1 -> Tilt Angle Controller/1(dcm_eb)
  Step5/1 -> Manual Switch5/1, Manual Switch3/1, Manual Switch4/1
  Tilt Angle Controller/2(deired_roll_rate_rad/s) -> Manual Switch4/2
  Manual Switch4/1 -> Saturation/1
  Manual Switch3/1 -> Saturation1/1
  Manual Switch5/1 -> Saturation5/1
  Tilt Angle Controller/1(Z) -> Vector Concatenate1/3
  [earth_linear_velocity] -> Zero-Order Hold7/1
  Demux3/2 -> Linear Velocity Controller/5(y_vel_current_earth)
  Demux3/1 -> Linear Velocity Controller/4(x_vel_current_earth)
  Demux3/3 -> Linear Velocity Controller/6(z_vel_current_earth)
  Zero-Order Hold7/1 -> Demux3/1
  Manual Switch9/1 -> Zero-Order Hold12/1
  Manual Switch11/1 -> Zero-Order Hold13/1
  Manual Switch10/1 -> Zero-Order Hold11/1
  Zero-Order Hold11/1 -> Linear Velocity Controller/1(x_vel_target_earth), To Workspace12/1
  Zero-Order Hold13/1 -> Linear Velocity Controller/3(z_vel_target_earth), To Workspace14/1
  Position Controller/1(x_vel_desired_earth) -> Saturation6/1
  Position Controller/2(y_vel_desired_earth) -> Saturation7/1
  Step6/1 -> Manual Switch10/1, Manual Switch9/1, Manual Switch11/1
  Linear Second-Order Actuator2/1 -> To Workspace15/1, Sum1/2  "Forces"
  Gravity and Drag Distrubance Calculation/6(FDz) -> ?  "force_drag_z"
  Gravity and Drag Distrubance Calculation/2(FGy) -> Vector Concatenate2/2  "force_gravity_y"
  Flight Kinematics/4 -> Math Function1/1, [dcm_body_earth]  "dcm_body_earth"
  Gravity and Drag Distrubance Calculation/1(FGx) -> Vector Concatenate2/1  "force_gravity_x"
  Math Function1/1 -> Gravity and Drag Distrubance Calculation/1(DCMeb)
  Flight Kinematics/5 -> Gravity and Drag Distrubance Calculation/2(Vb), [body_linear_velocity]  "body_linear_velocity"
  Gravity and Drag Distrubance Calculation/3(FGz) -> Vector Concatenate2/3  "force_gravity_z"
  Gravity and Drag Distrubance Calculation/4(FDx) -> ?  "force_drag_x"
  Gravity and Drag Distrubance Calculation/5(FDy) -> ?  "force_drag_y"
  Vector Concatenate2/1 -> Sum1/1
  Saturation6/1 -> Manual Switch10/2
  Saturation7/1 -> Manual Switch9/2
  Position Controller/3(z_vel_desired_earth) -> Manual Switch11/2
  Zero-Order Hold8/1 -> To Workspace1/1, Rate Controller/1(roll_rate_target)
  Zero-Order Hold9/1 -> To Workspace2/1, Rate Controller/2(pitch_rate_target)
  Zero-Order Hold10/1 -> To Workspace6/1, Rate Controller/3(yaw_rate_target)
  Zero-Order Hold19/1 -> Thrust Controller/1(desired_accel_x_earth), To Workspace3/1, Tilt Angle Controller/2(desired_accel_x_earth)
  Zero-Order Hold18/1 -> Thrust Controller/2(desired_accel_y_earth), To Workspace4/1, Tilt Angle Controller/3(desired_accel_y_earth)
  Zero-Order Hold17/1 -> Thrust Controller/3(desired_accel_z_earth), To Workspace5/1, Tilt Angle Controller/4(desired_accel_z_earth)
  Zero-Order Hold12/1 -> Linear Velocity Controller/2(y_vel_target_earth), To Workspace13/1
  Demux1/3 -> Tilt Angle Controller/5(current_Z_Force)
  Zero-Order Hold15/1 -> Demux1/1
  [body_forces] -> Zero-Order Hold15/1

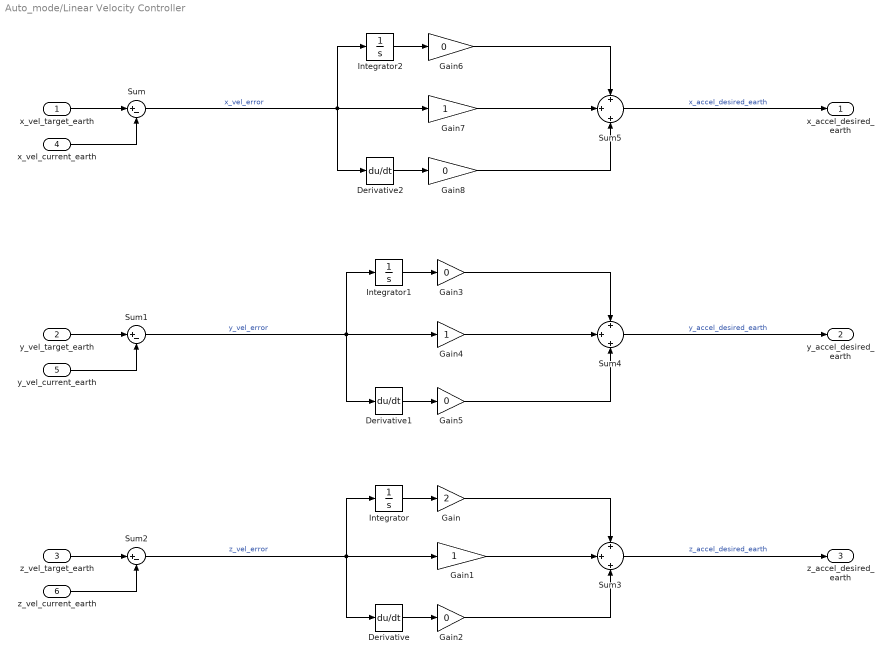
== system Auto_mode/Linear Velocity Controller ==
  x_vel_target_earth : Inport
  y_vel_target_earth : Inport  Port=2
  z_vel_target_earth : Inport  Port=3
  x_vel_current_earth : Inport  Port=4
  y_vel_current_earth : Inport  Port=5
  z_vel_current_earth : Inport  Port=6
  Derivative : Derivative
  Derivative1 : Derivative
  Derivative2 : Derivative
  Gain : Gain  Gain=2
  Gain1 : Gain
  Gain{2..3,5..6,8} (5 alike) : Gain  Gain=0
  Gain4 : Gain
  Gain7 : Gain
  Integrator : Integrator
  Integrator1 : Integrator
  Integrator2 : Integrator
  Sum : Sum  Inputs=|+-
  Sum1 : Sum  Inputs=|+-
  Sum2 : Sum  Inputs=|+-
  Sum3 : Sum  Inputs=+|+|+
  Sum4 : Sum  Inputs=+|+|+
  Sum5 : Sum  Inputs=+|+|+
  x_accel_desired_earth : Outport
  y_accel_desired_earth : Outport  Port=2
  z_accel_desired_earth : Outport  Port=3
  wires:
  x_vel_target_earth/1 -> Sum/1
  x_vel_current_earth/1 -> Sum/2
  y_vel_target_earth/1 -> Sum1/1
  y_vel_current_earth/1 -> Sum1/2
  z_vel_target_earth/1 -> Sum2/1
  z_vel_current_earth/1 -> Sum2/2
  Sum3/1 -> z_accel_desired_earth/1  "z_accel_desired_earth"
  Derivative/1 -> Gain2/1
  Gain2/1 -> Sum3/3
  Gain/1 -> Sum3/1
  Integrator/1 -> Gain/1
  Sum2/1 -> Integrator/1, Derivative/1, Gain1/1  "z_vel_error"
  Derivative1/1 -> Gain5/1
  Gain5/1 -> Sum4/3
  Gain4/1 -> Sum4/2
  Gain3/1 -> Sum4/1
  Integrator1/1 -> Gain3/1
  Sum1/1 -> Integrator1/1, Derivative1/1, Gain4/1  "y_vel_error"
  Sum4/1 -> y_accel_desired_earth/1  "y_accel_desired_earth"
  Derivative2/1 -> Gain8/1
  Gain8/1 -> Sum5/3
  Gain7/1 -> Sum5/2
  Gain6/1 -> Sum5/1
  Integrator2/1 -> Gain6/1
  Sum/1 -> Integrator2/1, Derivative2/1, Gain7/1  "x_vel_error"
  Sum5/1 -> x_accel_desired_earth/1  "x_accel_desired_earth"
  Gain1/1 -> Sum3/2

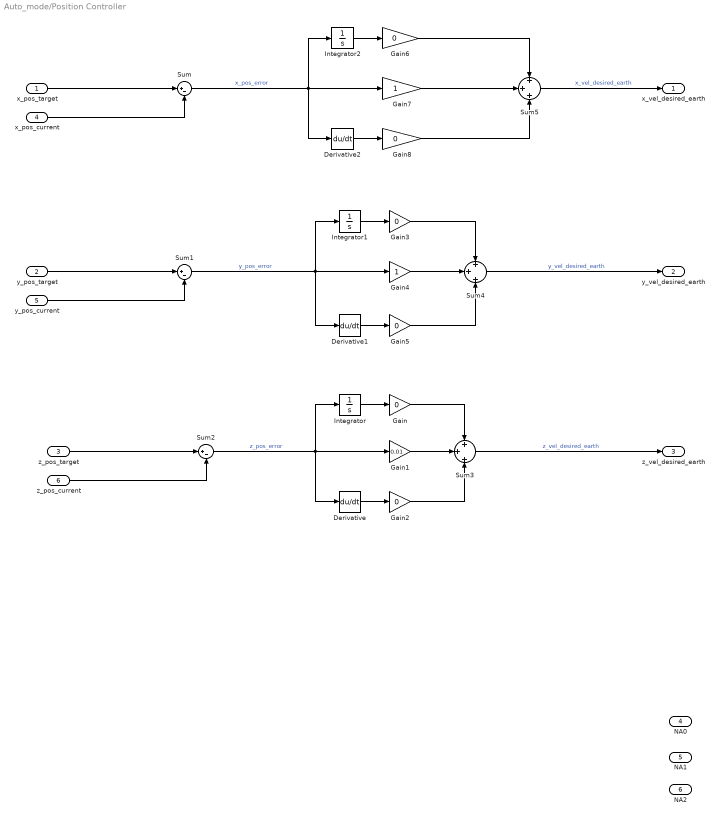
== system Auto_mode/Position Controller ==
  x_pos_target : Inport
  y_pos_target : Inport  Port=2
  z_pos_target : Inport  Port=3
  x_pos_current : Inport  Port=4
  y_pos_current : Inport  Port=5
  z_pos_current : Inport  Port=6
  Derivative : Derivative
  Derivative1 : Derivative
  Derivative2 : Derivative
  Gain{,2..3,5..6,8} (6 alike) : Gain  Gain=0
  Gain1 : Gain  Gain=0.01
  Gain4 : Gain
  Gain7 : Gain
  Integrator : Integrator
  Integrator1 : Integrator
  Integrator2 : Integrator
  Sum : Sum  Inputs=|+-
  Sum1 : Sum  Inputs=|+-
  Sum2 : Sum  Inputs=|+-
  Sum3 : Sum  Inputs=+|+|+
  Sum4 : Sum  Inputs=+|+|+
  Sum5 : Sum  Inputs=+|+|+
  x_vel_desired_earth : Outport
  y_vel_desired_earth : Outport  Port=2
  z_vel_desired_earth : Outport  Port=3
  NA0 : Outport  Port=4
  NA1 : Outport  Port=5
  NA2 : Outport  Port=6
  wires:
  x_pos_target/1 -> Sum/1
  x_pos_current/1 -> Sum/2
  y_pos_target/1 -> Sum1/1
  y_pos_current/1 -> Sum1/2
  z_pos_target/1 -> Sum2/1
  z_pos_current/1 -> Sum2/2
  Sum3/1 -> z_vel_desired_earth/1  "z_vel_desired_earth"
  Derivative/1 -> Gain2/1
  Gain2/1 -> Sum3/3
  Gain1/1 -> Sum3/2
  Gain/1 -> Sum3/1
  Integrator/1 -> Gain/1
  Sum2/1 -> Integrator/1, Derivative/1, Gain1/1  "z_pos_error"
  Derivative1/1 -> Gain5/1
  Gain5/1 -> Sum4/3
  Gain4/1 -> Sum4/2
  Gain3/1 -> Sum4/1
  Integrator1/1 -> Gain3/1
  Sum1/1 -> Integrator1/1, Derivative1/1, Gain4/1  "y_pos_error"
  Sum4/1 -> y_vel_desired_earth/1  "y_vel_desired_earth"
  Derivative2/1 -> Gain8/1
  Gain8/1 -> Sum5/3
  Gain7/1 -> Sum5/2
  Gain6/1 -> Sum5/1
  Integrator2/1 -> Gain6/1
  Sum/1 -> Integrator2/1, Derivative2/1, Gain7/1  "x_pos_error"
  Sum5/1 -> x_vel_desired_earth/1  "x_vel_desired_earth"

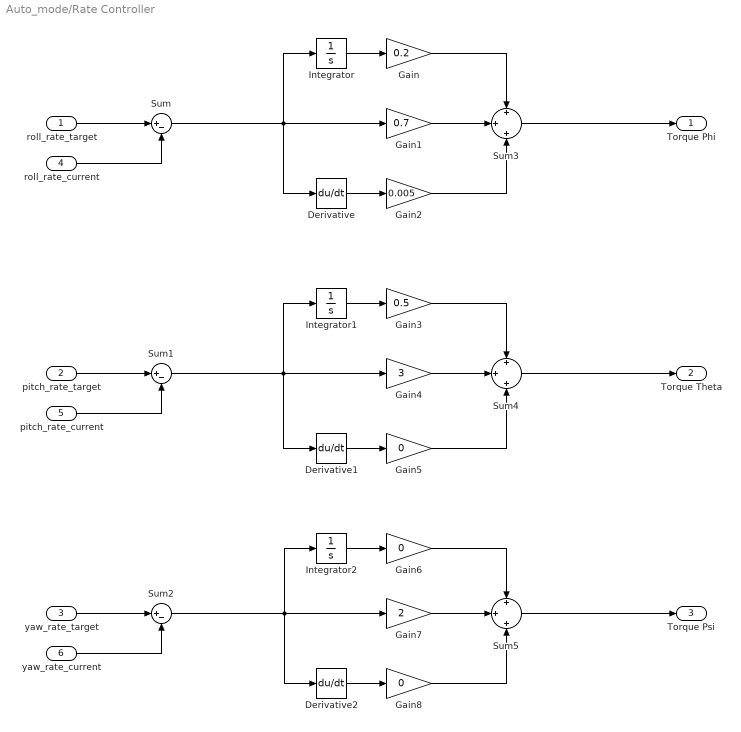
== system Auto_mode/Rate Controller ==
  roll_rate_target : Inport
  pitch_rate_target : Inport  Port=2
  yaw_rate_target : Inport  Port=3
  roll_rate_current : Inport  Port=4
  pitch_rate_current : Inport  Port=5
  yaw_rate_current : Inport  Port=6
  Derivative : Derivative
  Derivative1 : Derivative
  Derivative2 : Derivative
  Gain : Gain  Gain=0.2
  Gain1 : Gain  Gain=0.7
  Gain2 : Gain  Gain=0.005
  Gain3 : Gain  Gain=0.5
  Gain4 : Gain  Gain=3
  Gain5 : Gain  Gain=0
  Gain6 : Gain  Gain=0
  Gain7 : Gain  Gain=2
  Gain8 : Gain  Gain=0
  Integrator : Integrator
  Integrator1 : Integrator
  Integrator2 : Integrator
  Sum : Sum  Inputs=|+-
  Sum1 : Sum  Inputs=|+-
  Sum2 : Sum  Inputs=|+-
  Sum3 : Sum  Inputs=+|+|+
  Sum4 : Sum  Inputs=+|+|+
  Sum5 : Sum  Inputs=+|+|+
  Torque Phi : Outport
  Torque Theta : Outport  Port=2
  Torque Psi : Outport  Port=3
  wires:
  roll_rate_target/1 -> Sum/1
  roll_rate_current/1 -> Sum/2
  pitch_rate_target/1 -> Sum1/1
  pitch_rate_current/1 -> Sum1/2
  yaw_rate_target/1 -> Sum2/1
  yaw_rate_current/1 -> Sum2/2
  Sum4/1 -> Torque Theta/1
  Sum3/1 -> Torque Phi/1
  Derivative/1 -> Gain2/1
  Gain2/1 -> Sum3/3
  Gain1/1 -> Sum3/2
  Gain/1 -> Sum3/1
  Integrator/1 -> Gain/1
  Sum/1 -> Derivative/1, Integrator/1, Gain1/1
  Derivative1/1 -> Gain5/1
  Gain5/1 -> Sum4/3
  Gain4/1 -> Sum4/2
  Gain3/1 -> Sum4/1
  Integrator1/1 -> Gain3/1
  Sum1/1 -> Derivative1/1, Integrator1/1, Gain4/1
  Sum5/1 -> Torque Psi/1
  Derivative2/1 -> Gain8/1
  Gain8/1 -> Sum5/3
  Gain7/1 -> Sum5/2
  Gain6/1 -> Sum5/1
  Integrator2/1 -> Gain6/1
  Sum2/1 -> Gain7/1, Derivative2/1, Integrator2/1

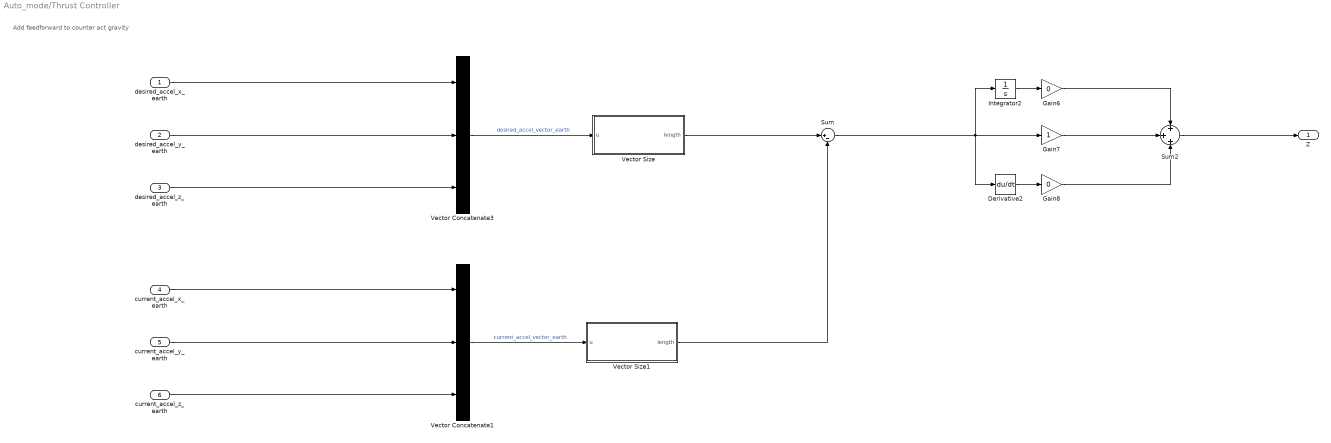
== system Auto_mode/Thrust Controller ==
  note: Add feedforward to counter act gravity
  desired_accel_x_earth : Inport
  desired_accel_y_earth : Inport  Port=2
  desired_accel_z_earth : Inport  Port=3
  current_accel_x_earth : Inport  Port=4
  current_accel_y_earth : Inport  Port=5
  current_accel_z_earth : Inport  Port=6
  Derivative2 : Derivative
  Gain6 : Gain  Gain=0
  Gain7 : Gain
  Gain8 : Gain  Gain=0
  Integrator2 : Integrator
  Sum : Sum  Inputs=|+-
  Sum2 : Sum  Inputs=+|+|+
  Vector Concatenate1 : Concatenate  NumInputs=3
  Vector Concatenate3 : Concatenate  NumInputs=3
  Vector Size : MATLAB Function  TreatAsAtomicUnit=on
  Vector Size1 : MATLAB Function  TreatAsAtomicUnit=on
  Z : Outport
  wires:
  desired_accel_x_earth/1 -> Vector Concatenate3/1
  desired_accel_y_earth/1 -> Vector Concatenate3/2
  desired_accel_z_earth/1 -> Vector Concatenate3/3
  Derivative2/1 -> Gain8/1
  Gain8/1 -> Sum2/3
  Gain7/1 -> Sum2/2
  Gain6/1 -> Sum2/1
  Integrator2/1 -> Gain6/1
  Sum/1 -> Integrator2/1, Derivative2/1, Gain7/1
  Sum2/1 -> Z/1
  Vector Size/1(length) -> Sum/1
  Vector Concatenate3/1 -> Vector Size/1(u)  "desired_accel_vector_earth"
  current_accel_x_earth/1 -> Vector Concatenate1/1
  current_accel_y_earth/1 -> Vector Concatenate1/2
  current_accel_z_earth/1 -> Vector Concatenate1/3
  Vector Concatenate1/1 -> Vector Size1/1(u)  "current_accel_vector_earth"
  Vector Size1/1(length) -> Sum/2

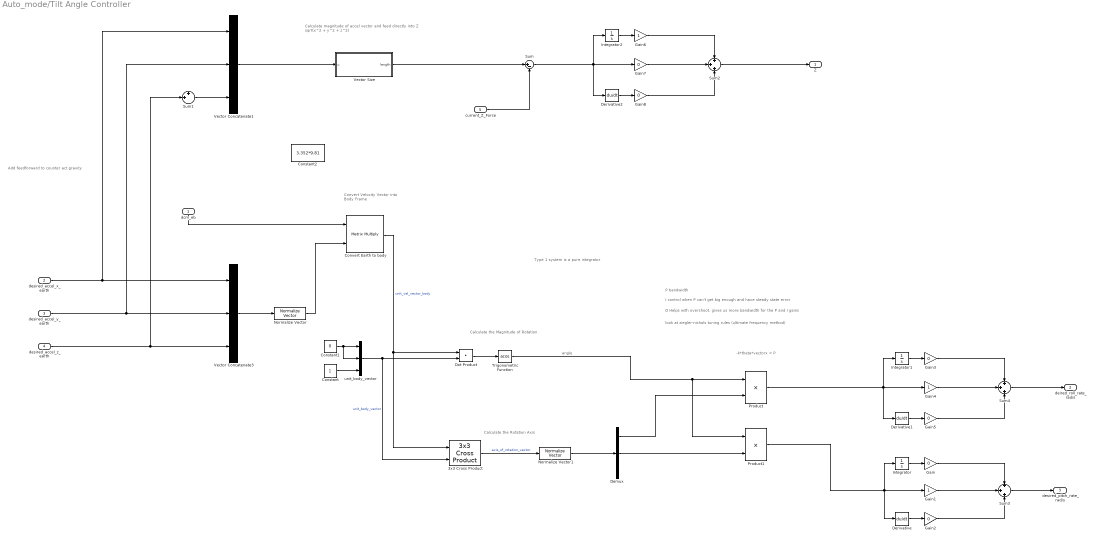
== system Auto_mode/Tilt Angle Controller ==
  note: Calculate magnitude of accel vector and feed directly into Z
      |
      | sqrt(x^2 + y^2 + z^2)
  note: D Helps with overshoot, gives us more bandwidth for the P and I gains
  note: I control when P can't get big enough and have steady state error
  note: P bandwidth
  note: look at ziegler-nichols tuning rules (ultimate frequency method)
  note: Type 1 system is a pure integrator
  note: angle
  note: -k*theta*vectorx = P
  note: Calculate the Rotation Axis
  note: Convert Velocity Vector into Body Frame
  note: Calculate the Magnitude of Rotation
  note: Add feedforward to counter act gravity
  dcm_eb : Inport
  desired_accel_x_earth : Inport  Port=2
  desired_accel_y_earth : Inport  Port=3
  desired_accel_z_earth : Inport  Port=4
  current_Z_Force : Inport  Port=5
  3x3 Cross Product : aerolibutil/3x3 Cross Product
  Constant : Constant
  Constant1 : Constant  Value=0
  Constant2 : Constant  Value=3.352*9.81
  Convert Earth to body : Product  Multiplication=Matrix(*)
  Demux : Demux  Outputs=3
  Derivative : Derivative
  Derivative1 : Derivative
  Derivative2 : Derivative
  Dot Product : DotProduct  InputSameDT=on  OutDataTypeStr=Inherit: Inherit via internal rule
  Gain{,2..3,5,7..8} (6 alike) : Gain  Gain=0
  Gain1 : Gain
  Gain4 : Gain
  Gain6 : Gain
  Integrator : Integrator
  Integrator1 : Integrator
  Integrator2 : Integrator
  Normalize Vector : vrlib/Utilities/Normalize Vector  maxzero=0
  Normalize Vector1 : vrlib/Utilities/Normalize Vector  maxzero=0
  Product : Product
  Product1 : Product
  Sum : Sum  Inputs=|+-
  Sum1 : Sum  Inputs=++|
  Sum2 : Sum  Inputs=+|+|+
  Sum3 : Sum  Inputs=+|+|+
  Sum4 : Sum  Inputs=+|+|+
  Trigonometric Function : Trigonometry  Operator=acos
  Vector Concatenate1 : Concatenate  NumInputs=3
  Vector Concatenate3 : Concatenate  NumInputs=3
  Vector Size : MATLAB Function  TreatAsAtomicUnit=on
  unit_body_vector : Concatenate  NumInputs=3
  Z : Outport
  deired_roll_rate_rad/s : Outport  Port=2
  desired_pitch_rate_rad/s : Outport  Port=3
  wires:
  desired_accel_x_earth/1 -> Vector Concatenate3/1, Vector Concatenate1/1
  desired_accel_y_earth/1 -> Vector Concatenate3/2, Vector Concatenate1/2
  desired_accel_z_earth/1 -> Sum1/2, Vector Concatenate3/3
  Vector Concatenate3/1 -> Normalize Vector/1
  Normalize Vector1/1 -> Demux/1
  Constant1/1 -> unit_body_vector/2, unit_body_vector/1
  Dot Product/1 -> Trigonometric Function/1
  Convert Earth to body/1 -> Dot Product/1, 3x3 Cross Product/1  "unit_vel_vector_body"
  Trigonometric Function/1 -> Product1/1, Product/1
  Constant/1 -> unit_body_vector/3
  dcm_eb/1 -> Convert Earth to body/1
  unit_body_vector/1 -> Dot Product/2, 3x3 Cross Product/2  "unit_body_vector"
  3x3 Cross Product/1 -> Normalize Vector1/1  "axis_of_rotation_vector"
  Normalize Vector/1 -> Convert Earth to body/2
  Sum1/1 -> Vector Concatenate1/3
  Vector Concatenate1/1 -> Vector Size/1(u)
  Sum3/1 -> desired_pitch_rate_rad/s/1
  Derivative/1 -> Gain2/1
  Gain2/1 -> Sum3/3
  Gain1/1 -> Sum3/2
  Gain/1 -> Sum3/1
  Integrator/1 -> Gain/1
  Derivative1/1 -> Gain5/1
  Gain5/1 -> Sum4/3
  Gain4/1 -> Sum4/2
  Gain3/1 -> Sum4/1
  Integrator1/1 -> Gain3/1
  Product/1 -> Integrator1/1, Derivative1/1, Gain4/1
  Product1/1 -> Derivative/1, Integrator/1, Gain1/1
  Sum4/1 -> deired_roll_rate_rad/s/1
  Demux/1 -> Product/2
  Demux/2 -> Product1/2
  Derivative2/1 -> Gain8/1
  Gain8/1 -> Sum2/3
  Gain7/1 -> Sum2/2
  Gain6/1 -> Sum2/1
  Integrator2/1 -> Gain6/1
  Sum/1 -> Integrator2/1, Derivative2/1, Gain7/1
  Sum2/1 -> Z/1
  Vector Size/1(length) -> Sum/1
  current_Z_Force/1 -> Sum/2

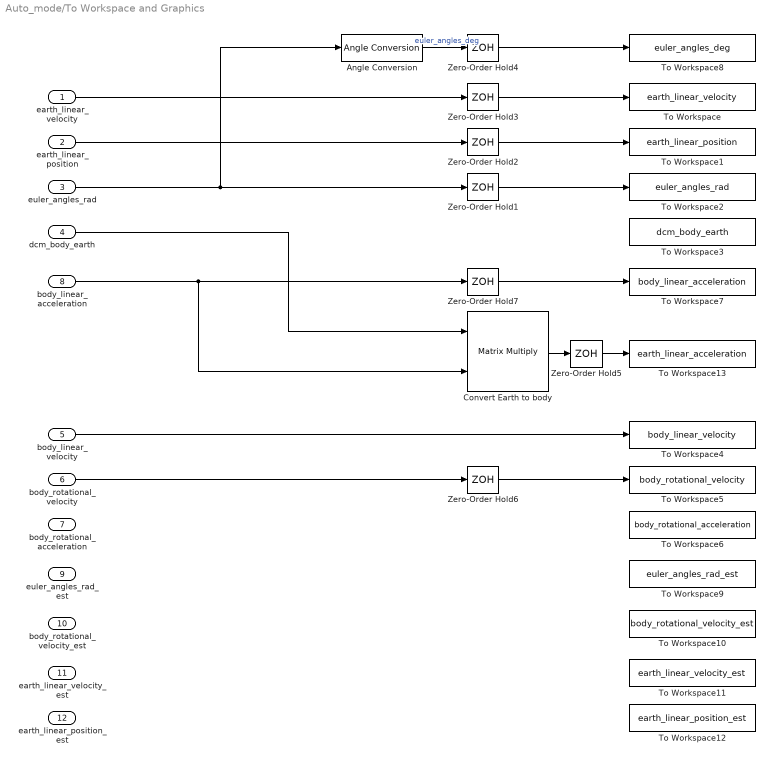
== system Auto_mode/To Workspace and Graphics ==
  earth_linear_velocity : Inport
  earth_linear_position : Inport  Port=2
  euler_angles_rad : Inport  Port=3
  dcm_body_earth : Inport  Port=4
  body_linear_velocity : Inport  Port=5
  body_rotational_velocity : Inport  Port=6
  body_rotational_acceleration : Inport  Port=7
  body_linear_acceleration : Inport  Port=8
  euler_angles_rad_est : Inport  Port=9
  body_rotational_velocity_est : Inport  Port=10
  earth_linear_velocity_est : Inport  Port=11
  earth_linear_position_est : Inport  Port=12
  Angle Conversion : aerolibconvert2/Angle Conversion  IU=rad  OU=deg
  Convert Earth to body : Product  Multiplication=Matrix(*)
  To Workspace : ToWorkspace  VariableName=earth_linear_velocity  SampleTime=-1
  To Workspace1 : ToWorkspace  VariableName=earth_linear_position  SampleTime=-1
  To Workspace10 : ToWorkspace  VariableName=body_rotational_velocity_est  SampleTime=-1
  To Workspace11 : ToWorkspace  VariableName=earth_linear_velocity_est  SampleTime=-1
  To Workspace12 : ToWorkspace  VariableName=earth_linear_position_est  SampleTime=-1
  To Workspace13 : ToWorkspace  VariableName=earth_linear_acceleration  SampleTime=-1
  To Workspace2 : ToWorkspace  VariableName=euler_angles_rad  SampleTime=-1
  To Workspace3 : ToWorkspace  VariableName=dcm_body_earth  SampleTime=-1
  To Workspace4 : ToWorkspace  VariableName=body_linear_velocity  SampleTime=-1
  To Workspace5 : ToWorkspace  VariableName=body_rotational_velocity  SampleTime=-1
  To Workspace6 : ToWorkspace  VariableName=body_rotational_acceleration  SampleTime=-1
  To Workspace7 : ToWorkspace  VariableName=body_linear_acceleration  SampleTime=-1
  To Workspace8 : ToWorkspace  VariableName=euler_angles_deg  SampleTime=-1
  To Workspace9 : ToWorkspace  VariableName=euler_angles_rad_est  SampleTime=-1
  Zero-Order Hold{1..7} (7 alike) : ZeroOrderHold  SampleTime=Ts
  wires:
  Angle Conversion/1 -> Zero-Order Hold4/1  "euler_angles_deg"
  euler_angles_rad/1 -> Zero-Order Hold1/1, Angle Conversion/1
  body_rotational_velocity/1 -> Zero-Order Hold6/1
  earth_linear_position/1 -> Zero-Order Hold2/1
  earth_linear_velocity/1 -> Zero-Order Hold3/1
  Zero-Order Hold6/1 -> To Workspace5/1
  Zero-Order Hold1/1 -> To Workspace2/1
  Zero-Order Hold2/1 -> To Workspace1/1
  Zero-Order Hold3/1 -> To Workspace/1
  Zero-Order Hold4/1 -> To Workspace8/1
  body_linear_velocity/1 -> To Workspace4/1
  Convert Earth to body/1 -> Zero-Order Hold5/1
  dcm_body_earth/1 -> Convert Earth to body/1
  body_linear_acceleration/1 -> Zero-Order Hold7/1, Convert Earth to body/2
  Zero-Order Hold5/1 -> To Workspace13/1
  Zero-Order Hold7/1 -> To Workspace7/1

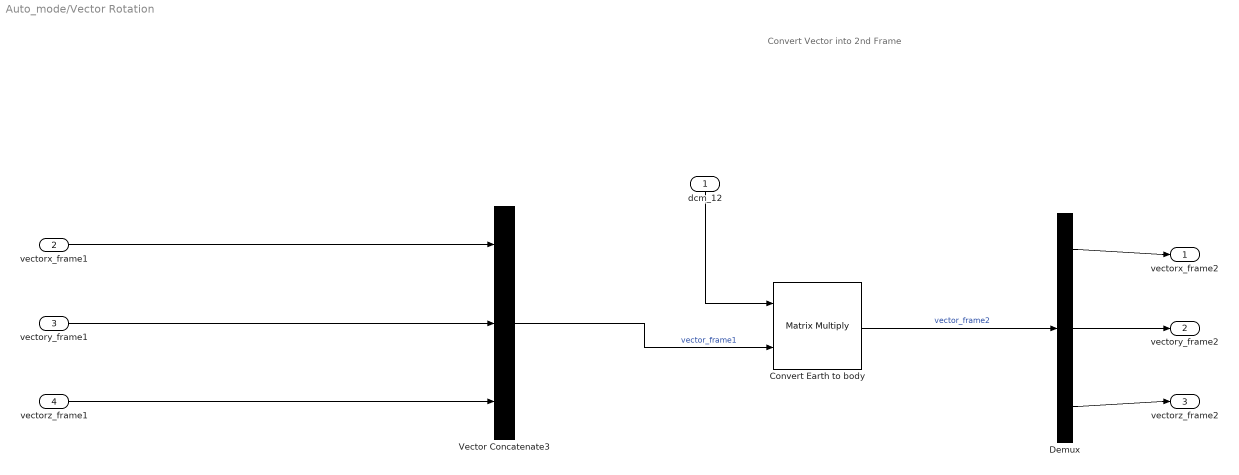
== system Auto_mode/Vector Rotation ==
  note: Convert Vector into 2nd Frame
  dcm_12 : Inport
  vectorx_frame1 : Inport  Port=2
  vectory_frame1 : Inport  Port=3
  vectorz_frame1 : Inport  Port=4
  Convert Earth to body : Product  Multiplication=Matrix(*)
  Demux : Demux  Outputs=3
  Vector Concatenate3 : Concatenate  NumInputs=3
  vectorx_frame2 : Outport
  vectory_frame2 : Outport  Port=2
  vectorz_frame2 : Outport  Port=3
  wires:
  vectorx_frame1/1 -> Vector Concatenate3/1
  vectory_frame1/1 -> Vector Concatenate3/2
  vectorz_frame1/1 -> Vector Concatenate3/3
  dcm_12/1 -> Convert Earth to body/1
  Vector Concatenate3/1 -> Convert Earth to body/2  "vector_frame1"
  Convert Earth to body/1 -> Demux/1  "vector_frame2"
  Demux/3 -> vectorz_frame2/1
  Demux/2 -> vectory_frame2/1
  Demux/1 -> vectorx_frame2/1

== matlab function Auto_mode/Thrust Controller/Vector Size ==
  data: u input; length output
function length = vectorLength(u)
%#codegen


length = sqrt( ((u(1))^2) + ((u(2))^2) + ((u(3))^2) );

== matlab function Auto_mode/Tilt Angle Controller/Vector Size ==
  data: u input; length output
function length = vectorLength(u)
%#codegen


length = sqrt( ((u(1))^2) + ((u(2))^2) + ((u(3))^2) );

== matlab function Auto_mode/Gravity and Drag Distrubance Calculation ==
  data: DCMeb input; FGx output; Vb input; FGy output; FGz output; FDx output; FDy output; FDz output
function [FGx, FGy, FGz, FDx, FDy, FDz] = gravityDragCalculation(DCMeb, Vb)
%   Gravity and Drag Calculations
%   Inputs
%   DCMbe = Direct Cosine Matrix, from earth to body
%   Vb = Linear Velocity, body frame
%   Outputs
%   FGa = Force of gravity in the 'a' axis, body frame
%   FDa = Force of drag in the 'a' axis, body frame

%Gravity Constants
mass = 3.352;
gravityForce_earth = [0, 0, (9.81*mass)];

%Drag Constants
airDensity = 1.1644; %wikipedia air density at 30 degrees C
dragCoefficient = 1.0; %SLADe
surfaceArea = [0.1, 0.5, 0.7]; 
Vbx = Vb(1);
Vby = Vb(2);
Vbz = Vb(3);

%Gravity Calculations
FG = gravityForce_earth * DCMeb;
FGx = FG(1);
FGy = FG(2);
FGz = FG(3);

% FGx = 0;
% FGy = 0;
% FGz = 0;

%Drag Calculations
% FDx = 0.5 * airDensity * (Vbx^2) * dragCoefficient * surfaceArea(1);
% FDy = 0.5 * airDensity * (Vby^2) * dragCoefficient * surfaceArea(2);
% FDz = 0.5 * airDensity * (Vbz^2) * dragCoefficient * surfaceArea(3);

 FDx = 0;
 FDy = 0;
 FDz = 0;


%% Trying some stupid stuff
% if Vbx > 0.000000000001
%     FDx = 0;
%     FDy = 0;
%     FDz = 0;
% else 
%     FDx = 0.5 * airDensity * (Vbx^2) * dragCoefficient * surfaceArea(1);
%     FDy = 0.5 * airDensity * (Vby^2) * dragCoefficient * surfaceArea(2);
%     FDz = 0.5 * airDensity * (Vbz^2) * dragCoefficient * surfaceArea(3);
% end

== matlab function Auto_mode/Thrust Controller/Vector Size1 ==
  data: u input; length output
function length = vectorLength(u)
%#codegen


length = sqrt( ((u(1))^2) + ((u(2))^2) + ((u(3))^2) );
